simulink model "manageILCTriggers_th"  (R2018a)
settings: Solver=VariableStepAuto  StartTime=0.0  StopTime=20  RelTol=1e-3
libraries: determineIterationPhase_ul x1, determineSimulationPhase_ul x1, manageILCTriggers_ul x1
settings Model: Creator=mitch  LastModifiedBy=mitch

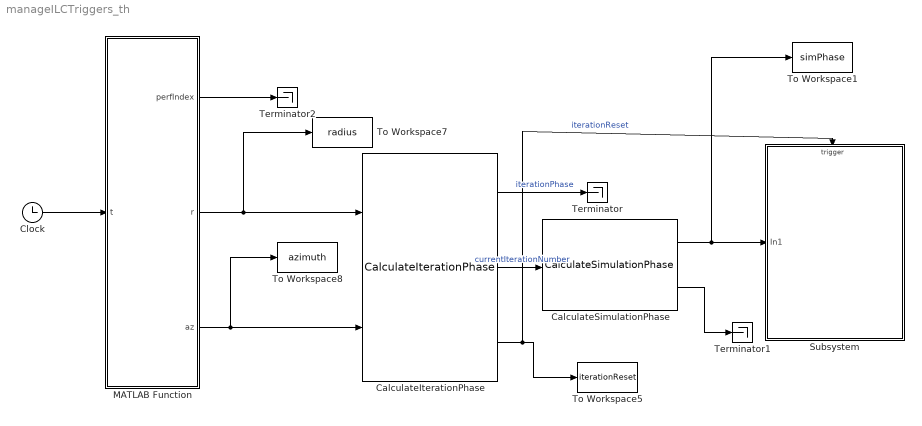
== system manageILCTriggers_th ==
  CalculateIterationPhase : determineIterationPhase_ul/CalculateIterationPhase
  CalculateSimulationPhase : determineSimulationPhase_ul/CalculateSimulationPhase
  Clock : Clock
  MATLAB Function : MATLAB Function  TreatAsAtomicUnit=on
  Subsystem : Subsystem
  Terminator : Terminator
  Terminator1 : Terminator
  Terminator2 : Terminator
  To Workspace1 : ToWorkspace  VariableName=simPhase  SaveFormat=Timeseries  SampleTime=-1
  To Workspace5 : ToWorkspace  VariableName=iterationReset  SaveFormat=Timeseries  SampleTime=-1
  To Workspace7 : ToWorkspace  VariableName=radius  SaveFormat=Timeseries  SampleTime=-1
  To Workspace8 : ToWorkspace  VariableName=azimuth  SaveFormat=Timeseries  SampleTime=-1
  wires:
  CalculateSimulationPhase/2 -> Terminator1/1
  CalculateIterationPhase/1 -> Terminator/1  "iterationPhase"
  MATLAB Function/3(az) -> To Workspace8/1, CalculateIterationPhase/2
  Clock/1 -> MATLAB Function/1(t)
  MATLAB Function/2(r) -> To Workspace7/1, CalculateIterationPhase/1
  CalculateIterationPhase/2 -> CalculateSimulationPhase/1  "currentIterationNumber"
  CalculateIterationPhase/3 -> Subsystem/Trigger, To Workspace5/1  "iterationReset"
  CalculateSimulationPhase/1 -> To Workspace1/1, Subsystem/1(In1)
  MATLAB Function/1(perfIndex) -> Terminator2/1

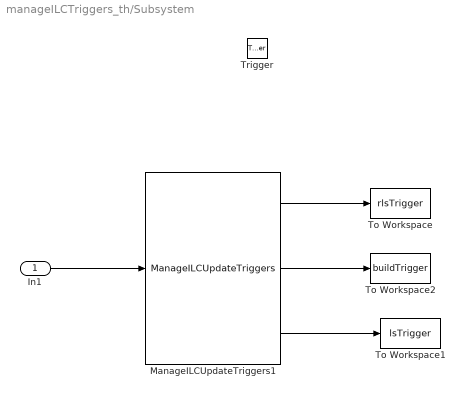
== system manageILCTriggers_th/Subsystem ==
  In1 : Inport
  Trigger : TriggerPort  VariantControl=Variant  PortDimensions=1
  ManageILCUpdateTriggers1 : manageILCTriggers_ul/ManageILCUpdateTriggers
  To Workspace : ToWorkspace  VariableName=rlsTrigger  SaveFormat=Timeseries  SampleTime=-1
  To Workspace1 : ToWorkspace  VariableName=lsTrigger  SaveFormat=Timeseries  SampleTime=-1
  To Workspace2 : ToWorkspace  VariableName=buildTrigger  SaveFormat=Timeseries  SampleTime=-1
  wires:
  In1/1 -> ManageILCUpdateTriggers1/1
  ManageILCUpdateTriggers1/2 -> To Workspace2/1
  ManageILCUpdateTriggers1/3 -> To Workspace1/1
  ManageILCUpdateTriggers1/1 -> To Workspace/1

== matlab function manageILCTriggers_th/MATLAB Function ==
  data: perfIndex output; r output; t input; az output
function [perfIndex,r,az] = fcn(t)
perfIndex = cos(2*pi*t+pi/5);
r = 70+35*sin(2*pi*t);
az = cos(2*pi*t);
end
